simulink model "part7_modebutton"  (R2022b)
settings: Solver=VariableStepAuto  StartTime=0.0  StopTime=10.0  RelTol=1e-3
settings Model: Creator=mingreico  LastModifiedBy=mingreico

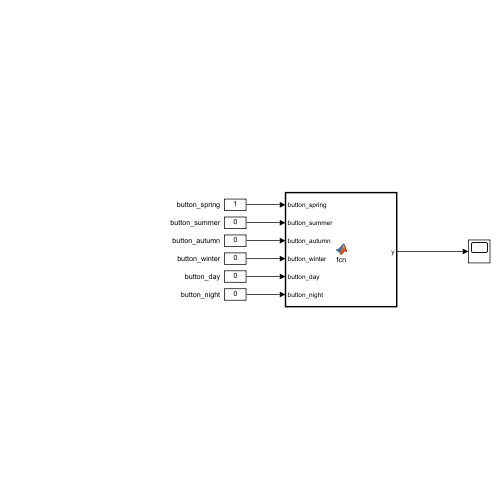
[thumbnail: Simulink's stored preview of the top-level diagram]
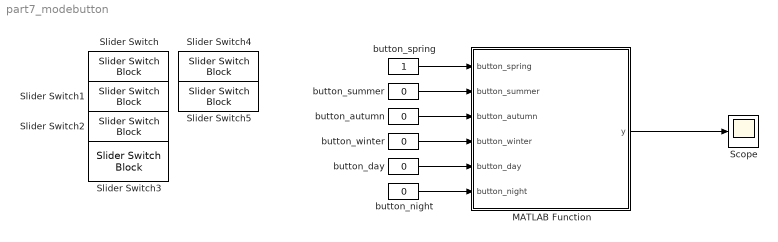
== system part7_modebutton ==
  MATLAB Function : MATLAB Function  TreatAsAtomicUnit=on
  Scope : Scope
  Slider Switch{,1..5} (6 alike) : SliderSwitchBlock
      settings: Values={{'Off', 'On'}, [0 1]}
  button_autumn : Constant  Value=0
  button_day : Constant  Value=0
  button_night : Constant  Value=0
  button_spring : Constant
  button_summer : Constant  Value=0
  button_winter : Constant  Value=0
  wires:
  button_spring/1 -> MATLAB Function/1(button_spring)
  button_summer/1 -> MATLAB Function/2(button_summer)
  button_autumn/1 -> MATLAB Function/3(button_autumn)
  button_winter/1 -> MATLAB Function/4(button_winter)
  button_day/1 -> MATLAB Function/5(button_day)
  button_night/1 -> MATLAB Function/6(button_night)
  MATLAB Function/1(y) -> Scope/1

== matlab function part7_modebutton/MATLAB Function ==
  data: button_spring input; y output; button_summer input; button_autumn input; button_winter input; button_day input; button_night input

function y = fcn(button_spring, button_summer, button_autumn, button_winter, button_day, button_night)
    persistent loadedData;
    timeVector = [0,1,2,3,4,5];
    % Default values
    default_season = 'spring';
    default_time = 'allday';
    if sum([button_spring, button_summer, button_autumn, button_winter] == 1) >1
        button_spring = 0;
        button_summer = 0;
        button_autumn = 0;
        button_winter = 0;
    end
    if isempty(loadedData)
        loadedData = load_default_data(default_season, default_time);
    elseif button_day || button_night||button_spring || button_summer || button_autumn || button_winter
        loadedData = load_data(button_spring, button_summer, button_autumn, button_winter, button_day, button_night);
    end
    y = timeseries(loadedData, timeVector);
end





function data = load_default_data(season, time)
    % Load default data or sequence
    % Modify this function to load the desired default data
    data = [1,2,3,3,2,1].';
end

function data = load_data(button_spring, button_summer, button_autumn, button_winter, button_day, button_night)
    % Load seasonal data or sequence based on the given season and time
    % Modify this function to load the desired seasonal data
    persistent loadData;
    allday_standard = [20,21,22,23,24,25].';
    % Check if no season button is pressed, default to spring
    if ~any([button_spring, button_summer, button_autumn, button_winter])
        button_spring = 1;
    end
    if button_day
        timefactor = 1.0;
    elseif button_night
        timefactor =2.0;
    else 
        timefactor = 0;
    end
    if button_spring
        if button_day||button_night
            loadData= [1,2,3,1,2,3].' *timefactor;
        else 
            loadData =allday_standard;
        end
    elseif button_summer
        if button_day||button_night
            loadData= [5,6,7,5,6,7].'* timefactor;
        else 
            loadData =allday_standard;
        end
    elseif button_autumn
         if button_day||button_night
            loadData= [10,11,12,10,11,12].' * timefactor;
        else 
            loadData =allday_standard;
         end
    elseif button_winter
        if button_day||button_night
            loadData= [15,16,17,15,16,17].' * timefactor;
        else 
            loadData =allday_standard;
        end
    else
        loadData = [0,0,0,0,0,0].';
    end
    data =loadData;
end
